simulink model "Type2_a"  (R2019a)
settings: Solver=VariableStepAuto  StartTime=0.0  StopTime=10.0  RelTol=1e-3
libraries: simulink x1
settings Model: Creator=admin  LastModifiedBy=admin

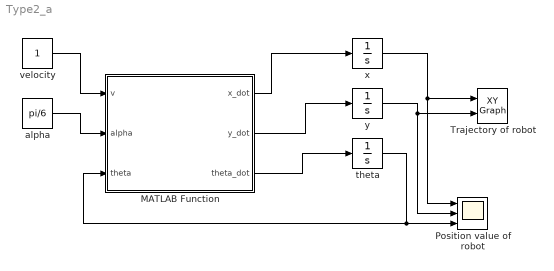
== system Type2_a ==
  MATLAB Function : MATLAB Function  TreatAsAtomicUnit=on
  Position value of robot : Scope  NumInputPorts=3
  Trajectory of robot : simulink/Sinks/XY Graph  xmin=-1  xmax=5  ymin=-1  ymax=7  st=-1
  alpha : Constant  Value=pi/6
  theta : Integrator
  velocity : Constant
  x : Integrator
  y : Integrator
  wires:
  velocity/1 -> MATLAB Function/1(v)
  alpha/1 -> MATLAB Function/2(alpha)
  MATLAB Function/1(x_dot) -> x/1
  MATLAB Function/2(y_dot) -> y/1
  MATLAB Function/3(theta_dot) -> theta/1
  theta/1 -> Position value of robot/3, MATLAB Function/3(theta)
  x/1 -> Position value of robot/1, Trajectory of robot/1
  y/1 -> Position value of robot/2, Trajectory of robot/2

== matlab function Type2_a/MATLAB Function ==
  data: v input; x_dot output; alpha input; theta input; y_dot output; theta_dot output
function [x_dot, y_dot, theta_dot] = tricycle_type_2(v, alpha, theta)
d = sqrt(3.1);
x_dot = v*cos(theta);
y_dot = v*sin(theta);
theta_dot = v/d*tan(alpha);
